simulink subsystem "WIN_MSGS_SENDER"  (R2022b)
settings: Solver=VariableStepAuto  StartTime=0.0  StopTime=10.0  RelTol=1e-3
settings Model: Creator=BEATOA  LastModifiedBy=BEATOA

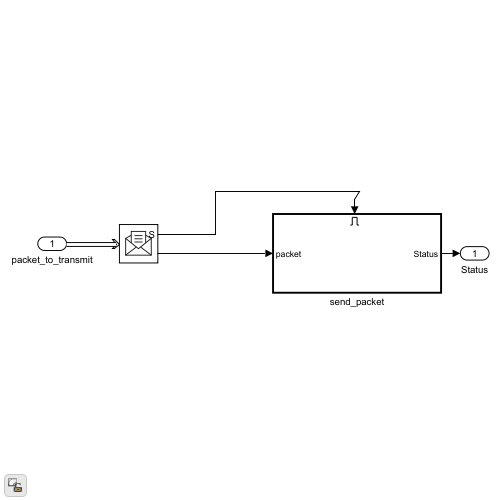
[thumbnail: Simulink's stored preview of the top-level diagram]
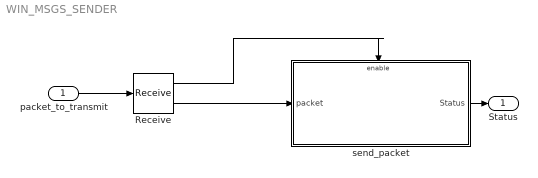
== system WIN_MSGS_SENDER ==
  packet_to_transmit : Inport
  Receive : Receive  InputPortMessageModes=m  UseInternalQueue=off  QueueOverwriting=on  QueueLength=64  ShowQueueStatus=on  ValueSourceWhenQueueIsEmpty=Use initial value  SampleTime=0.05
      settings: OutputPortMap=o0,o1
  send_packet : Subsystem
  Status : Outport
  wires:
  Receive/1 -> send_packet/Enable
  packet_to_transmit/1 -> Receive/1
  Receive/2 -> send_packet/1(packet)
  send_packet/1(Status) -> Status/1

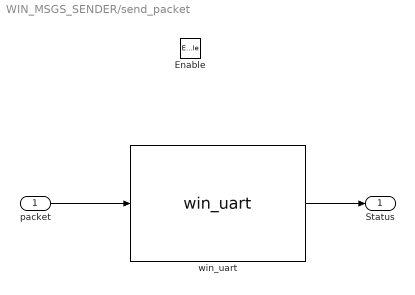
== system WIN_MSGS_SENDER/send_packet ==
  packet : Inport
  Enable : EnablePort
  win_uart : S-Function  FunctionName=win_uart  SFunctionDeploymentMode=off  EnableBusSupport=off
      mask Display:
      | port_label('input', 1, 'Packet');
      | port_label('output', 1, 'Status');
  Status : Outport  VectorParamsAs1DForOutWhenUnconnected=off
  wires:
  packet/1 -> win_uart/1
  win_uart/1 -> Status/1
